simulink model "my_robot_3_v2"  (R2013a)
settings: Solver=ode4  StartTime=0.0  StopTime=T  FixedStep=1/fs  RelTol=1e-3
values from neighbouring files (symbols this model uses):
  Kpf = Kpf/Wall.Ke    [Ejercicio3.m]
  Kpp = eye(robot.n) * 0.1 * (pi*fs)^2    [Ejercicio3.m]
  Kvf = 2*sqrt(Kpf)    [Ejercicio3.m]
  Kvp = 2*sqrt(Kpp)    [Ejercicio3.m]
  thetai = robot.ikine(Ti, [0, pi/2], [1 1 0 0 0 0])    [Ejercicio1.m]    (also in Ejercicio2.m; Ejercicio3.m)
settings Model: Creator=Juan Pablo  LastModifiedBy=root
settings DataIOCC: ExternalInput=[t, xSetpoint, FSetpoint]  LimitDataPoints=off  LoadExternalInput=on  SaveTime=off  OutputSaveName=q, x, Fe

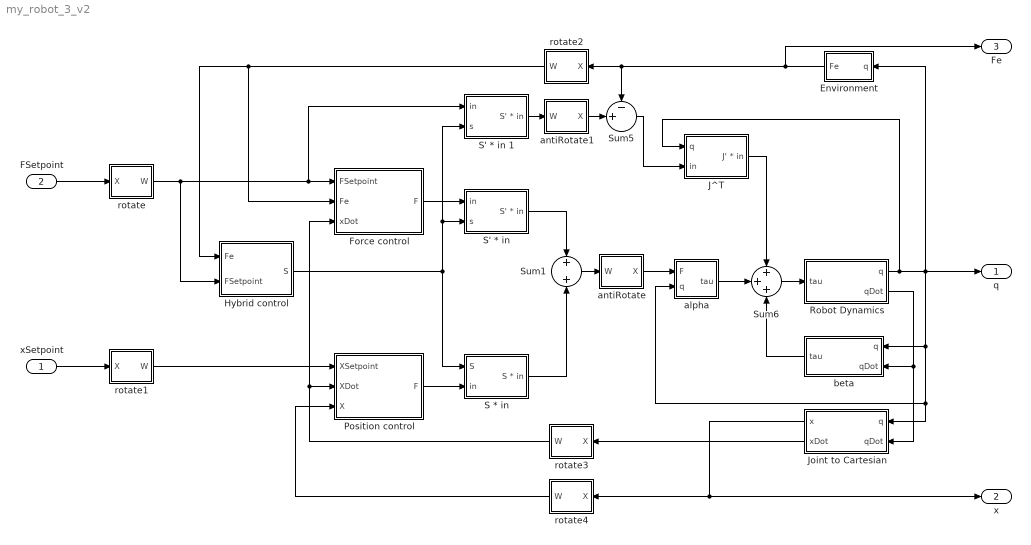
== system my_robot_3_v2 ==
  xSetpoint : Inport  PortDimensions=2
  FSetpoint : Inport  Port=2  PortDimensions=2
  Environment : Subsystem
  Force control : Subsystem
  Hybrid control : Subsystem
  J^T : Subsystem
  Joint to Cartesian : Subsystem
  Position control : Subsystem
  Robot Dynamics : Subsystem
  S * in : Subsystem
  "S' * in " : Subsystem
  S' * in 1 : Subsystem
  Sum1 : Sum  Inputs=+|+
  Sum5 : Sum  Inputs=-+|
  Sum6 : Sum  Inputs=+++
  alpha : Subsystem
  antiRotate : Subsystem
  antiRotate1 : Subsystem
  beta : Subsystem
  rotate : Subsystem
  rotate1 : Subsystem
  rotate2 : Subsystem
  rotate3 : Subsystem
  rotate4 : Subsystem
  q : Outport
  x : Outport  Port=2
  Fe : Outport  Port=3
  wires:
  Robot Dynamics/1(q) -> J^T/1(q), Environment/1(q), q/1, alpha/2(q), Joint to Cartesian/1(q), beta/1(q)
  Robot Dynamics/2(qDot) -> Joint to Cartesian/2(qDot), beta/2(qDot)
  Joint to Cartesian/1(x) -> rotate4/1(X), x/1
  Sum6/1 -> Robot Dynamics/1(tau)
  rotate/1(W) -> Hybrid control/2(FSetpoint), S' * in 1/1(in), Force control/1(FSetpoint)
  rotate3/1(W) -> Position control/2(XDot), Force control/3(xDot)
  antiRotate/1(X) -> alpha/1(F)
  Sum5/1 -> J^T/2(in)
  rotate1/1(W) -> Position control/1(XSetpoint)
  "S' * in "/1(S' * in) -> Sum1/1
  Force control/1(F) -> "S' * in "/1(in)
  S * in/1(S * in) -> Sum1/2
  Position control/1(F) -> S * in/2(in)
  alpha/1(tau) -> Sum6/2
  beta/1(tau) -> Sum6/3
  Hybrid control/1(S) -> S * in/1(S), "S' * in "/2(s), S' * in 1/2(s)
  FSetpoint/1 -> rotate/1(X)
  xSetpoint/1 -> rotate1/1(X)
  Sum1/1 -> antiRotate/1(W)
  Environment/1(Fe) -> Fe/1, Sum5/1, rotate2/1(X)
  rotate2/1(W) -> Force control/2(Fe), Hybrid control/1(Fe)
  Joint to Cartesian/2(xDot) -> rotate3/1(X)
  rotate4/1(W) -> Position control/3(X)
  J^T/1(J' * in) -> Sum6/1
  antiRotate1/1(X) -> Sum5/2
  S' * in 1/1(S' * in) -> antiRotate1/1(W)

== system my_robot_3_v2/Environment ==
  q : Inport
  Environment force : M-S-Function  FunctionName=environment  Parameters=robot, Wall
  Fe : Outport
  wires:
  q/1 -> Environment force/1
  Environment force/1 -> Fe/1

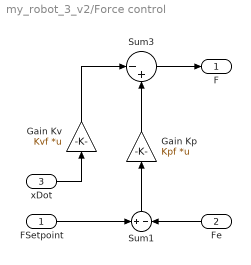
== system my_robot_3_v2/Force control ==
  FSetpoint : Inport
  Fe : Inport  Port=2
  xDot : Inport  Port=3
  Gain Kp : Gain  Gain=Kpf  Multiplication=Matrix(K*u)
  Gain Kv : Gain  Gain=Kvf  Multiplication=Matrix(K*u)
  Sum1 : Sum  Inputs=+|-
  Sum3 : Sum  Inputs=|-+
  F : Outport
  wires:
  Fe/1 -> Sum1/2
  FSetpoint/1 -> Sum1/1
  Sum1/1 -> Gain Kp/1
  Sum3/1 -> F/1
  Gain Kp/1 -> Sum3/2
  xDot/1 -> Gain Kv/1
  Gain Kv/1 -> Sum3/1

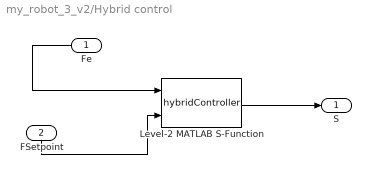
== system my_robot_3_v2/Hybrid control ==
  Fe : Inport
  FSetpoint : Inport  Port=2
  Level-2 MATLAB S-Function : M-S-Function  FunctionName=hybridController
  S : Outport
  wires:
  FSetpoint/1 -> Level-2 MATLAB S-Function/2
  Fe/1 -> Level-2 MATLAB S-Function/1
  Level-2 MATLAB S-Function/1 -> S/1

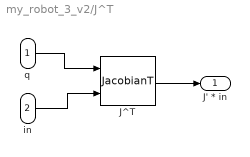
== system my_robot_3_v2/J^T ==
  q : Inport
  in : Inport  Port=2
  J^T : M-S-Function  FunctionName=JacobianT  Parameters=robot
  J' * in : Outport
  wires:
  q/1 -> J^T/1
  J^T/1 -> J' * in/1
  in/1 -> J^T/2

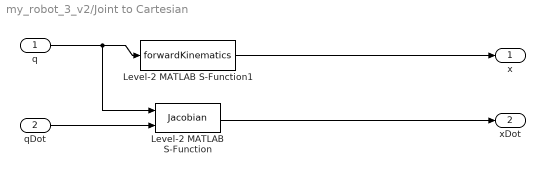
== system my_robot_3_v2/Joint to Cartesian ==
  q : Inport
  qDot : Inport  Port=2
  Level-2 MATLAB S-Function : M-S-Function  FunctionName=Jacobian  Parameters=robot
  Level-2 MATLAB S-Function1 : M-S-Function  FunctionName=forwardKinematics  Parameters=robot
  x : Outport
  xDot : Outport  Port=2
  wires:
  q/1 -> Level-2 MATLAB S-Function1/1, Level-2 MATLAB S-Function/1
  qDot/1 -> Level-2 MATLAB S-Function/2
  Level-2 MATLAB S-Function/1 -> xDot/1
  Level-2 MATLAB S-Function1/1 -> x/1

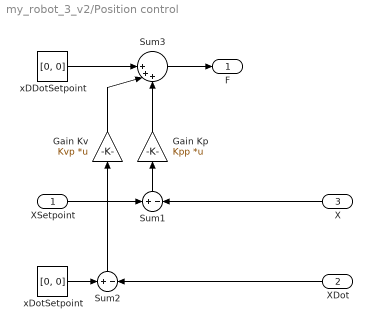
== system my_robot_3_v2/Position control ==
  XSetpoint : Inport
  XDot : Inport  Port=2
  X : Inport  Port=3
  Gain Kp : Gain  Gain=Kpp  Multiplication=Matrix(K*u)
  Gain Kv : Gain  Gain=Kvp  Multiplication=Matrix(K*u)
  Sum1 : Sum  Inputs=+|-
  Sum2 : Sum  Inputs=+|-
  Sum3 : Sum  Inputs=||+++
  xDDotSetpoint : Constant  Value=[0, 0]
  xDotSetpoint : Constant  Value=[0, 0]
  F : Outport
  wires:
  X/1 -> Sum1/2
  Gain Kv/1 -> Sum3/2
  Sum2/1 -> Gain Kv/1
  XDot/1 -> Sum2/2
  xDotSetpoint/1 -> Sum2/1
  Sum1/1 -> Gain Kp/1
  xDDotSetpoint/1 -> Sum3/1
  Sum3/1 -> F/1
  Gain Kp/1 -> Sum3/3
  XSetpoint/1 -> Sum1/1

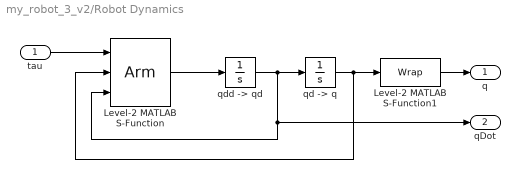
== system my_robot_3_v2/Robot Dynamics ==
  tau : Inport
  Level-2 MATLAB S-Function : M-S-Function  FunctionName=Arm  Parameters=probot
  Level-2 MATLAB S-Function1 : M-S-Function  FunctionName=Wrap  Parameters=robot
  "qd -> q" : Integrator  InitialCondition=thetai
  "qdd -> qd" : Integrator
  q : Outport
  qDot : Outport  Port=2
  wires:
  Level-2 MATLAB S-Function/1 -> "qdd -> qd"/1
  "qdd -> qd"/1 -> Level-2 MATLAB S-Function/3, qDot/1, "qd -> q"/1
  "qd -> q"/1 -> Level-2 MATLAB S-Function/2, Level-2 MATLAB S-Function1/1
  tau/1 -> Level-2 MATLAB S-Function/1
  Level-2 MATLAB S-Function1/1 -> q/1

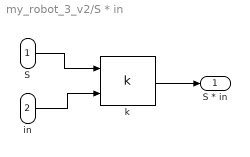
== system my_robot_3_v2/S * in ==
  S : Inport
  in : Inport  Port=2
  "k " : M-S-Function  FunctionName=k
  S * in : Outport
  wires:
  S/1 -> "k "/1
  "k "/1 -> S * in/1
  in/1 -> "k "/2

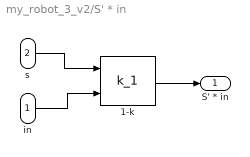
== system my_robot_3_v2/S' * in  ==
  in : Inport
  s : Inport  Port=2
  1-k : M-S-Function  FunctionName=k_1
  S' * in : Outport
  wires:
  s/1 -> 1-k/1
  1-k/1 -> S' * in/1
  in/1 -> 1-k/2

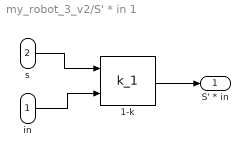
== system my_robot_3_v2/S' * in 1 ==
  in : Inport
  s : Inport  Port=2
  1-k : M-S-Function  FunctionName=k_1
  S' * in : Outport
  wires:
  s/1 -> 1-k/1
  1-k/1 -> S' * in/1
  in/1 -> 1-k/2

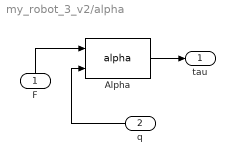
== system my_robot_3_v2/alpha ==
  F : Inport
  q : Inport  Port=2
  Alpha : M-S-Function  FunctionName=alpha  Parameters=robot
  tau : Outport
  wires:
  q/1 -> Alpha/2
  F/1 -> Alpha/1
  Alpha/1 -> tau/1

== system my_robot_3_v2/antiRotate ==
  W : Inport
  rotate : M-S-Function  FunctionName=antiRotate  Parameters=Wall
  X : Outport
  wires:
  W/1 -> rotate/1
  rotate/1 -> X/1

== system my_robot_3_v2/antiRotate1 ==
  W : Inport
  rotate : M-S-Function  FunctionName=antiRotate  Parameters=Wall
  X : Outport
  wires:
  W/1 -> rotate/1
  rotate/1 -> X/1

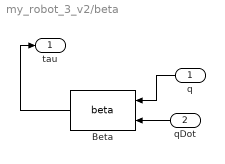
== system my_robot_3_v2/beta ==
  q : Inport
  qDot : Inport  Port=2
  Beta : M-S-Function  FunctionName=beta  Parameters=robot
  tau : Outport
  wires:
  Beta/1 -> tau/1
  q/1 -> Beta/1
  qDot/1 -> Beta/2

== system my_robot_3_v2/rotate ==
  X : Inport
  rotate : M-S-Function  FunctionName=rotate  Parameters=Wall
  W : Outport
  wires:
  X/1 -> rotate/1
  rotate/1 -> W/1

== system my_robot_3_v2/rotate1 ==
  X : Inport
  rotate : M-S-Function  FunctionName=rotate  Parameters=Wall
  W : Outport
  wires:
  X/1 -> rotate/1
  rotate/1 -> W/1

== system my_robot_3_v2/rotate2 ==
  X : Inport
  rotate : M-S-Function  FunctionName=rotate  Parameters=Wall
  W : Outport
  wires:
  X/1 -> rotate/1
  rotate/1 -> W/1

== system my_robot_3_v2/rotate3 ==
  X : Inport
  rotate : M-S-Function  FunctionName=rotate  Parameters=Wall
  W : Outport
  wires:
  X/1 -> rotate/1
  rotate/1 -> W/1

== system my_robot_3_v2/rotate4 ==
  X : Inport
  rotate : M-S-Function  FunctionName=rotate  Parameters=Wall
  W : Outport
  wires:
  X/1 -> rotate/1
  rotate/1 -> W/1
